simulink model "sm_cable_space_manipulator"  (R2021b)
settings: Solver=ode45  StartTime=0.0  StopTime=13  MaxStep=0.2  RelTol=1e-4
model workspace: external: MATLAB File sm_cable_space_manipulator_parameters.m (data not in the file)
undefined symbols (not defined in the file or in its folder): JointPlate1, LeftInnerJointPlate, LinkPulley, LinkSolid, PulleyClampSolid, RightInnerJointPlate, sigbuilder_block, SinglePulleyClampSolid, SlidingPulleyClamp, smiData, SpreaderPulley, SpreaderSolid, SpreaderSupportSolid, X, Y, Z
libraries: sm_lib x502, nesl_utility x26
(part 14 of 14)

== matlab function sm_cable_space_manipulator/Manipulator1/360Deg_Joint_System/JointPlate1/BeltContactPointApproximationWhenPackaged/BeltContactPointMovement ==
  data: movement_signal output; pulleyanglediff input
function movement_signal = fcn(pulleyanglediff)
% Approximating the Belt-Contact Point Movement using additonal pulleys
% like 'BeltContactP1'.
% This fcn takes in the difference between the 
% pulley angles of 'BeltContactP1' pulley.
% The 'BeltContactP1' pulley is on a motion actuated prismatic joint along
% the direction of the Link.
% When the mechanism is packaged, the cable/belt entering and 
% leaving this pulley has a non zero angle (AngleDiff < 0) and the
% 'BeltContactP1' pulley is fixed at the approximated position (near the spreader).
% When the mechanism is opening, based on the AngleDiff range, the
% 'BeltContactP1' pulley Prismatic moves it to an approximated position
% (Near the Motor).

persistent i;
if isempty(i)
    i = 1;
    movement_signal = 2.45;
else
    if (pulleyanglediff>-2 && pulleyanglediff~=0 && i == 1)
        movement_signal = 2.45;
    else
        movement_signal = 2.45-i*0.01;
        
        i = i+1;
    end

end

== matlab function sm_cable_space_manipulator/Manipulator1/360Deg_Joint_System/JointPlate2/BeltContactPointApproximationWhenPackaged1/BeltContactPointMovement ==
  data: movement_signal output; pulleyanglediff input
function movement_signal = fcn(pulleyanglediff)
% Approximating the Belt-Contact Point Movement using additonal pulleys
% like 'BeltContactP1'.
% This fcn takes in the difference between the 
% pulley angles of 'BeltContactP1' pulley.
% The 'BeltContactP1' pulley is on a motion actuated prismatic joint along
% the direction of the Link.
% When the mechanism is packaged, the cable/belt entering and 
% leaving this pulley has a non zero angle (AngleDiff < 0) and the
% 'BeltContactP1' pulley is fixed at the approximated position (near the spreader).
% When the mechanism is opening, based on the AngleDiff range, the
% 'BeltContactP1' pulley Prismatic moves it to an approximated position
% (Near the Motor).

persistent i;
if isempty(i)
    i = 1;
    movement_signal = 2.45;
else
    if (pulleyanglediff>-2 && pulleyanglediff~=0 && i == 1)
        movement_signal = 2.45;
    else
        movement_signal = 2.45-i*0.01;
        
        i = i+1;
    end

end

== matlab function sm_cable_space_manipulator/Manipulator2/360Deg_Joint_System/JointPlate1/BeltContactPointApproximationWhenPackaged/BeltContactPointMovement ==
  data: movement_signal output; pulleyanglediff input
function movement_signal = fcn(pulleyanglediff)
% Approximating the Belt-Contact Point Movement using additonal pulleys
% like 'BeltContactP1'.
% This fcn takes in the difference between the 
% pulley angles of 'BeltContactP1' pulley.
% The 'BeltContactP1' pulley is on a motion actuated prismatic joint along
% the direction of the Link.
% When the mechanism is packaged, the cable/belt entering and 
% leaving this pulley has a non zero angle (AngleDiff < 0) and the
% 'BeltContactP1' pulley is fixed at the approximated position (near the spreader).
% When the mechanism is opening, based on the AngleDiff range, the
% 'BeltContactP1' pulley Prismatic moves it to an approximated position
% (Near the Motor).

persistent i;
if isempty(i)
    i = 1;
    movement_signal = 2.45;
else
    if (pulleyanglediff>-2 && pulleyanglediff~=0 && i == 1)
        movement_signal = 2.45;
    else
        movement_signal = 2.45-i*0.01;
        
        i = i+1;
    end

end

== matlab function sm_cable_space_manipulator/Manipulator2/360Deg_Joint_System/JointPlate2/BeltContactPointApproximationWhenPackaged1/BeltContactPointMovement ==
  data: movement_signal output; pulleyanglediff input
function movement_signal = fcn(pulleyanglediff)
% Approximating the Belt-Contact Point Movement using additonal pulleys
% like 'BeltContactP1'.
% This fcn takes in the difference between the 
% pulley angles of 'BeltContactP1' pulley.
% The 'BeltContactP1' pulley is on a motion actuated prismatic joint along
% the direction of the Link.
% When the mechanism is packaged, the cable/belt entering and 
% leaving this pulley has a non zero angle (AngleDiff < 0) and the
% 'BeltContactP1' pulley is fixed at the approximated position (near the spreader).
% When the mechanism is opening, based on the AngleDiff range, the
% 'BeltContactP1' pulley Prismatic moves it to an approximated position
% (Near the Motor).

persistent i;
if isempty(i)
    i = 1;
    movement_signal = 2.45;
else
    if (pulleyanglediff>-2 && pulleyanglediff~=0 && i == 1)
        movement_signal = 2.45;
    else
        movement_signal = 2.45-i*0.01;
        
        i = i+1;
    end

end

== matlab function sm_cable_space_manipulator/Motion Inputs/ManipBaseRev_q ==
  data: y output; t input
function y = fcn(t)
% S curve motion profile.
L = 2.5;
k = 1;
t0 = 4.5/2;
y = L/(1+exp(-k*(t-t0)))-L/(1+exp(-k*(0-t0)));
end

== matlab function sm_cable_space_manipulator/Motion Inputs/ManipPulleyMotion_q ==
  data: t input; y output
function y = fcn(t)
% S curve motion profile.
if t>=0 && t<0.5
    y = 0;
elseif t>=0.5 && t < 4.8
  
    k = 3;
    t0 = (4.79+0.5)/2;
    L = 3;
    y = L/(1+exp(-k*(t-t0)))-L/(1+exp(-k*(0.5-t0)));
    
elseif t>=4.8 && t<5
    L = 3;
    k = 3;
    t0 = (4.79+0.5)/2;
    y = L/(1+exp(-k*(4.79-t0)))-L/(1+exp(-k*(0.5-t0))); 
elseif t>=5 && t<13
    L = -2;
    k = 3;
    t0 = (6+12.9)/2;
    y = L/(1+exp(-k*(t-t0)))+3/(1+exp(-3*(4.79-(4.79+0.5)/2)))-3/(1+exp(-3*(0.5-(4.79+0.5)/2)));
        
else
    L = -2;
    k = 3;
    t0 = (6+13.9)/2;
    t = 13.9;
    y = L/(1+exp(-k*(t-t0)))+3/(1+exp(-3*(4.79-(4.79+0.5)/2)))-3/(1+exp(-3*(0.5-(4.79+0.5)/2)));
end
